simulink model "genericAW"  (Simulink 8.5)
settings: Solver=ode5  SolverMode=SingleTasking  StartTime=0.0  StopTime=tstop  FixedStep=tstep  RelTol=1e-3  AbsTol=1e-6
values from neighbouring files (symbols this model uses):
  Ac = [A1 B1; zeros(2,5) zeros(2,2)]    [BTTmissile_sim.m]
  Ap = [-0.818   -0.999    0.349 ... (first row only)    [BTTmissile_sim.m]
  AW = AWfull2    [BTTmissile_sim.m]    (also in fullorder_ct_polef.m = ss(Ap+Bp*F,Bp,[F; Cp+Dp*F],[zeros(m,m); Dp]); fullorder_ctf.m = ss(Ap+Bp*F,Bp,[F; Cp+Dp*F],[zeros(m,m); Dp]))
  baru = ubar    (= 8)    [BTTmissile_sim.m]
  Bc = -[zeros(5,2) ; eye(2)]    [BTTmissile_sim.m]
  Bcr = -Bc    [BTTmissile_sim.m]
  Bp = [0.147    0.012 ... (first row only)    [BTTmissile_sim.m]
  Bpd = zeros(3,2)    [BTTmissile_sim.m]
  Cc = [0.86 8.54 -1.71 43.91 1.12 0 0 ... (first row only)    [BTTmissile_sim.m]
  Cp = [1   0   0 ... (first row only)    [BTTmissile_sim.m]
  Dc = -zeros(2,2)    [BTTmissile_sim.m]
  Dcr = -Dc    [BTTmissile_sim.m]
  Dp = zeros(2,2)    [BTTmissile_sim.m]
  Dpd = zeros(2,2)    [BTTmissile_sim.m]
  p = size(Cp,1)    [fullorder_ct_polef.m]    (also in fullorder_ctf.m; lureconsensus.m = size(C,1))
undefined symbols (not defined in the file or in its folder): m, nd, nr
settings Model: Creator=mct6  LastModifiedBy=mct6  ExtModeTrigMode=oneshot  ExtModeArmWhenConnect=off  ExtModeAutoUpdateStatusClock=off
settings DataIOCC: LimitDataPoints=off  SaveOutput=off  SignalLoggingName=sigsOut
settings OptimizationCC: BooleanDataType=off  ExpressionDepthLimit=128  InitFltsAndDblsToZero=on
settings DebuggingCC: AlgebraicLoopMsg=none  SaveWithParameterizedLinksMsg=none  SignalResolutionControl=TryResolveAllWithWarning  MultiTaskDSMMsg=warning  MultiTaskCondExecSysMsg=none  FcnCallInpInsideContextMsg=UseLocalSettings  StateNameClashWarn=none
settings HardwareCC: TargetUnknown=on
settings GRTTargetCC: TargetFcnLib=ansi_tfl_tmw.mat  ModelReferenceCompliant=off  MatFileLogging=off

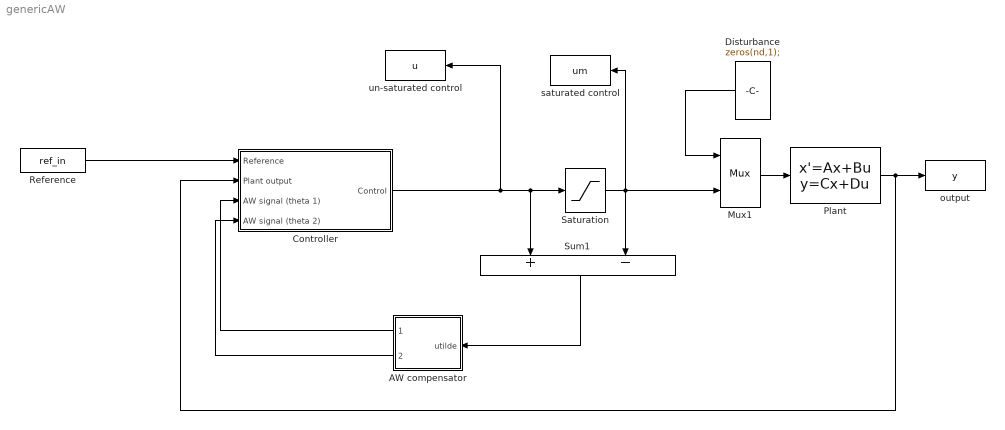
== system genericAW ==
  AW compensator : Subsystem
  Controller : Subsystem
  Disturbance : Constant  Value=zeros(nd,1);
  Mux1 : Mux  Inputs=[nd m]
  Plant : StateSpace  A=Ap  B=[Bpd Bp]  C=Cp  D=[Dpd Dp]  X0=0
  Reference : FromWorkspace  VariableName=ref_in  SampleTime=0
  Saturation : Saturate  UpperLimit=baru  LowerLimit=-baru
  Sum1 : Sum  Inputs=+-  SaturateOnIntegerOverflow=on  InputSameDT=on  OutDataTypeStr=Inherit: Same as first input
  output : ToWorkspace  VariableName=y  SaveFormat=Structure With Time  SampleTime=-1
  saturated control : ToWorkspace  VariableName=um  SaveFormat=Structure With Time  SampleTime=-1
  un-saturated control : ToWorkspace  VariableName=u  SaveFormat=Structure With Time  SampleTime=-1
  wires:
  Controller/1(Control) -> Saturation/1, Sum1/1, un-saturated control/1
  Plant/1 -> output/1, Controller/2(Plant output)
  Saturation/1 -> Sum1/2, Mux1/2, saturated control/1
  Sum1/1 -> AW compensator/1(utilde)
  AW compensator/2(theta 2) -> Controller/4(AW signal (theta 2))
  AW compensator/1(theta 1) -> Controller/3(AW signal (theta 1))
  Reference/1 -> Controller/1(Reference)
  Mux1/1 -> Plant/1
  Disturbance/1 -> Mux1/1

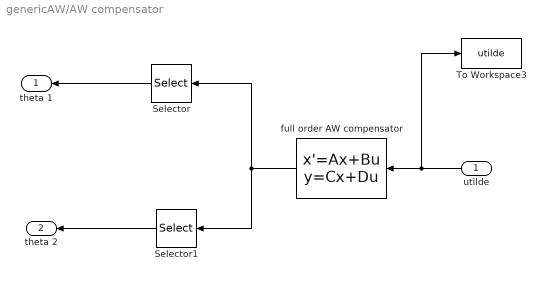
== system genericAW/AW compensator ==
  utilde : Inport
  Selector : Selector  InputPortWidth=m+p  Indices=[1:m]
  Selector1 : Selector  InputPortWidth=m+p  Indices=[m+1:m+p]
  To Workspace3 : ToWorkspace  VariableName=utilde  SaveFormat=Structure With Time  SampleTime=-1
  full order AW compensator : StateSpace  A=AW.a  B=AW.b  C=AW.c  D=AW.d  X0=0
  theta 1 : Outport  InitialOutput=0
  theta 2 : Outport  Port=2  InitialOutput=0
  wires:
  utilde/1 -> full order AW compensator/1, To Workspace3/1
  full order AW compensator/1 -> Selector/1, Selector1/1
  Selector/1 -> theta 1/1
  Selector1/1 -> theta 2/1

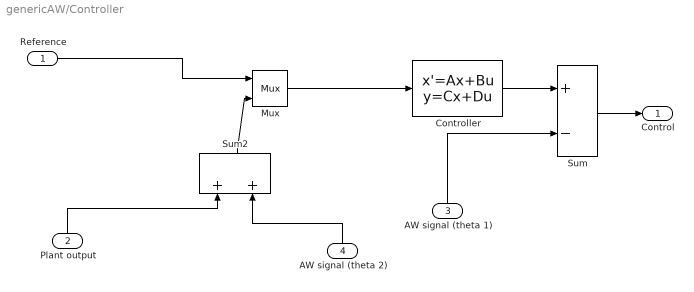
== system genericAW/Controller ==
  Reference : Inport
  Plant output : Inport  Port=2
  AW signal (theta 1) : Inport  Port=3
  AW signal (theta 2) : Inport  Port=4
  Controller : StateSpace  A=Ac  B=[Bcr Bc]  C=Cc  D=[Dcr Dc]  X0=0
  Mux : Mux  Inputs=[nr p]
  Sum : Sum  Inputs=+-  SaturateOnIntegerOverflow=on  InputSameDT=on  OutDataTypeStr=Inherit: Same as first input
  Sum2 : Sum  SaturateOnIntegerOverflow=on  InputSameDT=on  OutDataTypeStr=Inherit: Same as first input
  Control : Outport
  wires:
  Mux/1 -> Controller/1
  Sum2/1 -> Mux/2
  Plant output/1 -> Sum2/1
  Reference/1 -> Mux/1
  Controller/1 -> Sum/1
  Sum/1 -> Control/1
  AW signal (theta 1)/1 -> Sum/2
  AW signal (theta 2)/1 -> Sum2/2
